simulink model "ctrl_tilt_16b"  (R2016b)
settings: Solver=FixedStepDiscrete  StartTime=0.0  StopTime=25  FixedStep=0.001  RelTol=1e-3  EnableMultiTasking=on
values from neighbouring files (symbols this model uses):
  Par_mdlQuad = mdl_quadrotor_par()    [ctrl_tilt_16b_init.m]
libraries: arduinolib x1
settings Model: ExtModeTrigDuration=2  Creator=Nu  LastModifiedBy=Nu
settings OptimizationCC: MaxStackSize=64
settings DebuggingCC: ParameterTunabilityLossMsg=error
settings HardwareCC: ProdBitPerInt=16  ProdBitPerPointer=16  ProdBitPerSizeT=16  ProdBitPerPtrDiffT=16  ProdLargestAtomicFloat=None  ProdWordSize=8  ProdHWDeviceType=Atmel->AVR
settings RTWCC: SystemTargetFile=ert.tlc  HardwareBoard=Arduino Nano 3.0  TLCOptions=-aInlineSetEventsForThisBaseRateFcn=TLC_FALSE -aSuppressMultiTaskScheduler=TLC_FALSE -aRateBasedStepFcn=1  TemplateMakefile=ert_default_tmf  Description=Embedded Coder  GenerateReport=on  Toolchain=Arduino AVR  BuildConfiguration=Faster Runs  IncludeHyperlinkInReport=on  LaunchReport=on  GenerateTraceInfo=on  GenerateTraceReport=on  GenerateTraceReportSl=on  GenerateTraceReportSf=on  GenerateTraceReportEml=on
settings CodeAppCC: ForceParamTrailComments=on  IgnoreCustomStorageClasses=off  OperatorAnnotations=on  SimulinkDataObjDesc=on  SFDataObjDesc=on  MATLABFcnDesc=on  InsertBlockDesc=on  MATLABSourceComments=on
settings ERTTargetCC: SupportContinuousTime=on  SupportVariableSizeSignals=on

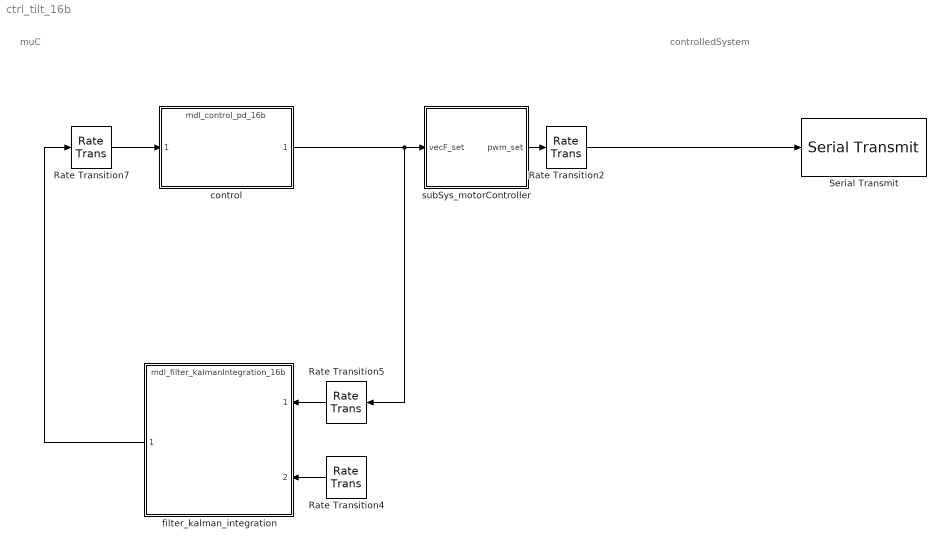
== system ctrl_tilt_16b ==
  note: controlledSystem
  note: muC
  Rate Transition2 : RateTransition
  Rate Transition4 : RateTransition  OutPortSampleTime=Par_filterKalman.T
  Rate Transition5 : RateTransition  X0=Par_mdlQuad.F0*ones(4,1)
  Rate Transition7 : RateTransition
  Serial Transmit : arduinolib/Serial Transmit  portNumber=0  blockPlatform=arduino
  control : ModelReference  ModelNameDialog=mdl_control_pd_16b.slx  SimulationMode=Normal  ModelReferenceVersion=1.284
  filter_kalman_integration : ModelReference  ModelNameDialog=mdl_filter_kalmanIntegration_16b.slx  SimulationMode=Normal  ModelReferenceVersion=1.174
  subSys_motorController : Subsystem
  wires:
  ? -> Rate Transition4/1
  Rate Transition2/1 -> Serial Transmit/1
  Rate Transition4/1 -> filter_kalman_integration/2
  filter_kalman_integration/1 -> Rate Transition7/1
  Rate Transition5/1 -> filter_kalman_integration/1
  subSys_motorController/1(pwm_set) -> Rate Transition2/1
  control/1 -> subSys_motorController/1(vecF_set), Rate Transition5/1
  Rate Transition7/1 -> control/1

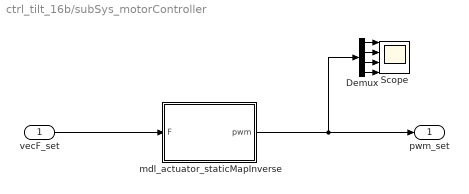
== system ctrl_tilt_16b/subSys_motorController ==
  vecF_set : Inport
  Demux : Demux
  Scope : Scope  NumInputPorts=4
  mdl_actuator_staticMapInverse : MATLAB Function  TreatAsAtomicUnit=on
  pwm_set : Outport
  wires:
  vecF_set/1 -> mdl_actuator_staticMapInverse/1(F)
  mdl_actuator_staticMapInverse/1(pwm) -> Demux/1, pwm_set/1
  Demux/1 -> Scope/1
  Demux/2 -> Scope/2
  Demux/3 -> Scope/3
  Demux/4 -> Scope/4

== matlab function ctrl_tilt_16b/subSys_motorController/mdl_actuator_staticMapInverse ==
  data: F input; pwm output
function pwm = fcn( F )

pwm = mdl_actuator_staticMapInverse( F );
